simulink model "simulateAIModel_R2025a"  (R2025a)
settings: Solver=VariableStepAuto  StopTime=15000
undefined symbols (not defined in the file or in its folder): quantizedNet
libraries: dlconvfclib x9, dlactivationlib x4, dlpoolinglib x1, dlinputlayernormlib x1
settings Model: Creator=wenzheli  LastModifiedBy=wenzheli

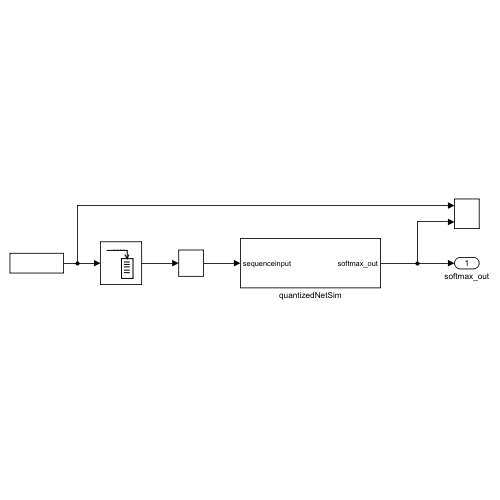
[thumbnail: Simulink's stored preview of the top-level diagram]
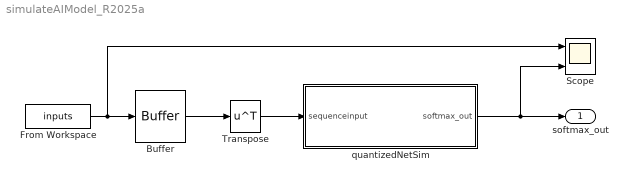
== system simulateAIModel_R2025a ==
  Buffer : Buffer  N=5000  V=64  OutputFrames=off
  From Workspace : FromWorkspace  VariableName=inputs  SampleTime=1
  Scope : Scope  NumInputPorts=2
      settings: Title=Classification Probability  ActiveDisplayYMinimum=-0.25749358226609853  ActiveDisplayYMaximum=1.1288244571901096
  Transpose : Math  Operator=transpose
  quantizedNetSim : Subsystem
  softmax_out : Outport
  wires:
  From Workspace/1 -> Scope/1, Buffer/1
  Buffer/1 -> Transpose/1
  Transpose/1 -> quantizedNetSim/1(sequenceinput)
  quantizedNetSim/1(softmax_out) -> Scope/2, softmax_out/1

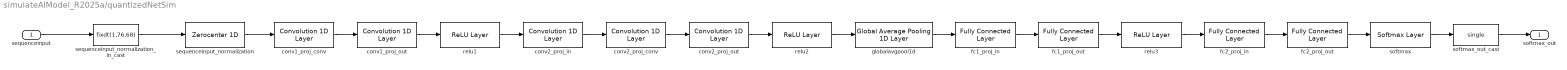
== system simulateAIModel_R2025a/quantizedNetSim ==
  sequenceinput : Inport  PortDimensions="[1  5000]"
  conv1_proj_conv : dlconvfclib/Convolution 1D Layer  Layer=quantizedNet.Layers(2)  PermuteDims=[2 1]  OutMin=[]  OutMax=[]  OutDataTypeStr=fixdt(1,8,2)  RndMeth=Nearest  SaturateOnIntegerOverflow=on  WeightsDataTypeStr=fixdt(1,8,8)  WeightsMin=[]  WeightsMax=[]  BiasDataTypeStr=fixdt(1,32,11)  BiasMin=[]  BiasMax=[]  AccumDataTypeStr=fixdt(1,32,11)  InternalRndMeth=Nearest  InternalSaturateOnIntegerOverflow=off  SampleTime=-1
      settings: DataFormat=CT
  conv1_proj_out : dlconvfclib/Convolution 1D Layer  Layer=quantizedNet.Layers(3)  PermuteDims=[2 1]  OutMin=[]  OutMax=[]  OutDataTypeStr=fixdt(1,8,3)  RndMeth=Nearest  SaturateOnIntegerOverflow=on  WeightsDataTypeStr=fixdt(1,8,7)  WeightsMin=[]  WeightsMax=[]  BiasDataTypeStr=fixdt(1,32,9)  BiasMin=[]  BiasMax=[]  AccumDataTypeStr=fixdt(1,32,9)  InternalRndMeth=Nearest  InternalSaturateOnIntegerOverflow=off  SampleTime=-1
      settings: DataFormat=CT
  conv2_proj_conv : dlconvfclib/Convolution 1D Layer  Layer=quantizedNet.Layers(6)  PermuteDims=[2 1]  OutMin=[]  OutMax=[]  OutDataTypeStr=fixdt(1,8,0)  RndMeth=Nearest  SaturateOnIntegerOverflow=on  WeightsDataTypeStr=fixdt(1,8,7)  WeightsMin=[]  WeightsMax=[]  BiasDataTypeStr=fixdt(1,32,10)  BiasMin=[]  BiasMax=[]  AccumDataTypeStr=fixdt(1,32,10)  InternalRndMeth=Nearest  InternalSaturateOnIntegerOverflow=off  SampleTime=-1
      settings: DataFormat=CT
  conv2_proj_in : dlconvfclib/Convolution 1D Layer  Layer=quantizedNet.Layers(5)  PermuteDims=[2 1]  OutMin=[]  OutMax=[]  OutDataTypeStr=fixdt(1,8,3)  RndMeth=Nearest  SaturateOnIntegerOverflow=on  WeightsDataTypeStr=fixdt(1,8,7)  WeightsMin=[]  WeightsMax=[]  BiasDataTypeStr=fixdt(1,32,10)  BiasMin=[]  BiasMax=[]  AccumDataTypeStr=fixdt(1,32,10)  InternalRndMeth=Nearest  InternalSaturateOnIntegerOverflow=off  SampleTime=-1
      settings: DataFormat=CT
  conv2_proj_out : dlconvfclib/Convolution 1D Layer  Layer=quantizedNet.Layers(7)  PermuteDims=[2 1]  OutMin=[]  OutMax=[]  OutDataTypeStr=fixdt(1,8,0)  RndMeth=Nearest  SaturateOnIntegerOverflow=on  WeightsDataTypeStr=fixdt(1,8,7)  WeightsMin=[]  WeightsMax=[]  BiasDataTypeStr=fixdt(1,32,7)  BiasMin=[]  BiasMax=[]  AccumDataTypeStr=fixdt(1,32,7)  InternalRndMeth=Nearest  InternalSaturateOnIntegerOverflow=off  SampleTime=-1
      settings: DataFormat=CT
  fc1_proj_in : dlconvfclib/Fully Connected Layer  Layer=quantizedNet.Layers(10)  OutMin=[]  OutMax=[]  OutDataTypeStr=fixdt(1,8,4)  RndMeth=Nearest  SaturateOnIntegerOverflow=on  WeightsDataTypeStr=fixdt(1,8,7)  WeightsMin=[]  WeightsMax=[]  BiasDataTypeStr=fixdt(1,32,10)  BiasMin=[]  BiasMax=[]  AccumDataTypeStr=fixdt(1,32,10)  AccumMin=[]  AccumMax=[]  InternalRndMeth=Nearest  InternalSaturateOnIntegerOverflow=off  SampleTime=-1
      settings: DataFormat=C
  fc1_proj_out : dlconvfclib/Fully Connected Layer  Layer=quantizedNet.Layers(11)  OutMin=[]  OutMax=[]  OutDataTypeStr=fixdt(1,8,5)  RndMeth=Nearest  SaturateOnIntegerOverflow=on  WeightsDataTypeStr=fixdt(1,8,7)  WeightsMin=[]  WeightsMax=[]  BiasDataTypeStr=fixdt(1,32,11)  BiasMin=[]  BiasMax=[]  AccumDataTypeStr=fixdt(1,32,11)  AccumMin=[]  AccumMax=[]  InternalRndMeth=Nearest  InternalSaturateOnIntegerOverflow=off  SampleTime=-1
      settings: DataFormat=C
  fc2_proj_in : dlconvfclib/Fully Connected Layer  Layer=quantizedNet.Layers(13)  OutMin=[]  OutMax=[]  OutDataTypeStr=fixdt(1,8,2)  RndMeth=Nearest  SaturateOnIntegerOverflow=on  WeightsDataTypeStr=fixdt(1,8,7)  WeightsMin=[]  WeightsMax=[]  BiasDataTypeStr=fixdt(1,32,12)  BiasMin=[]  BiasMax=[]  AccumDataTypeStr=fixdt(1,32,12)  AccumMin=[]  AccumMax=[]  InternalRndMeth=Nearest  InternalSaturateOnIntegerOverflow=off  SampleTime=-1
      settings: DataFormat=C
  fc2_proj_out : dlconvfclib/Fully Connected Layer  Layer=quantizedNet.Layers(14)  OutMin=[]  OutMax=[]  OutDataTypeStr=fixdt(1,8,2)  RndMeth=Nearest  SaturateOnIntegerOverflow=on  WeightsDataTypeStr=fixdt(1,8,7)  WeightsMin=[]  WeightsMax=[]  BiasDataTypeStr=fixdt(1,32,9)  BiasMin=[]  BiasMax=[]  AccumDataTypeStr=fixdt(1,32,9)  AccumMin=[]  AccumMax=[]  InternalRndMeth=Nearest  InternalSaturateOnIntegerOverflow=off  SampleTime=-1
      settings: DataFormat=C
  globalavgpool1d : dlpoolinglib/Global Average Pooling 1D Layer  Layer=quantizedNet.Layers(9)  InputSize="[3  5000]"  OutMin=[]  OutMax=[]  OutDataTypeStr=fixdt(1,8,3)  RndMeth=Nearest  SaturateOnIntegerOverflow=on  AccumDataTypeStr=fixdt(1,32,0)  NumPoolingElementsDataTypeStr=fixdt(0,32,0)  NumPoolingElementsMin=[]  NumPoolingElementsMax=[]  InternalRndMeth=Nearest  InternalSaturateOnIntegerOverflow=on  SampleTime=-1
      settings: DataFormat=CT
  relu1 : dlactivationlib/ReLU Layer  OutMin=[]  OutMax=[]  OutDataTypeStr=fixdt(1,8,3)  SampleTime=-1
  relu2 : dlactivationlib/ReLU Layer  OutMin=[]  OutMax=[]  OutDataTypeStr=fixdt(1,8,0)  SampleTime=-1
  relu3 : dlactivationlib/ReLU Layer  OutMin=[]  OutMax=[]  OutDataTypeStr=fixdt(1,8,5)  SampleTime=-1
  sequenceinput_normalization : dlinputlayernormlib/Zerocenter 1D  Layer=quantizedNet.Layers(1)  OutMin=[]  OutMax=[]  OutDataTypeStr=fixdt(1,8,3)  RndMeth=Nearest  SaturateOnIntegerOverflow=on  MeanDataTypeStr=fixdt(0,8,68)  MeanMin=[]  MeanMax=[]  AccumDataTypeStr=fixdt(1,76,68)  InternalRndMeth=Nearest  InternalSaturateOnIntegerOverflow=off  SampleTime=-1
      settings: DataFormat=CT
  sequenceinput_normalization_in_cast : DataTypeConversion  OutDataTypeStr=fixdt(1,76,68)  RndMeth=Nearest
  softmax : dlactivationlib/Softmax Layer  ApproximationMethod=Lookup  OutMin=[]  OutMax=[]  OutDataTypeStr=fixdt(0,8,8)  RndMeth=Nearest  SaturateOnIntegerOverflow=on  AccumDataTypeStr=fixdt(0,32,16)  InternalRndMeth=Nearest  InternalSaturateOnIntegerOverflow=on  SampleTime=-1
      settings: DataFormat=C
  softmax_out_cast : DataTypeConversion  OutDataTypeStr=single  SaturateOnIntegerOverflow=off  RndMeth=Floor
  softmax_out : Outport
  wires:
  globalavgpool1d/1 -> fc1_proj_in/1
  softmax_out_cast/1 -> softmax_out/1
  conv2_proj_out/1 -> relu2/1
  fc2_proj_out/1 -> softmax/1
  relu2/1 -> globalavgpool1d/1
  conv2_proj_in/1 -> conv2_proj_conv/1
  relu1/1 -> conv2_proj_in/1
  conv1_proj_out/1 -> relu1/1
  sequenceinput_normalization_in_cast/1 -> sequenceinput_normalization/1
  fc2_proj_in/1 -> fc2_proj_out/1
  conv2_proj_conv/1 -> conv2_proj_out/1
  sequenceinput_normalization/1 -> conv1_proj_conv/1
  conv1_proj_conv/1 -> conv1_proj_out/1
  sequenceinput/1 -> sequenceinput_normalization_in_cast/1
  fc1_proj_in/1 -> fc1_proj_out/1
  relu3/1 -> fc2_proj_in/1
  softmax/1 -> softmax_out_cast/1
  fc1_proj_out/1 -> relu3/1
